simulink model "Q0107tsmc_egtsmc_egftsmc_final_sensitivity"  (R2024b)
settings: Solver=ode4  StartTime=0.0  StopTime=12  FixedStep=0.01  RelTol=1e-3  EnableMultiTasking=on
model workspace (MAT data in the model file):
  A1 = 0.0190784648009
  A2 = 0.089786568484
  B1 = 2.58582251419
  B2 = 0.593361860386
  Count = 20
  I1 = 0.276
  I2 = 0.0235
  I3 = 0.0235
  L1 = 0.5
  L2 = 0.4
  Lp1d = 0.49
  Lp2d = 0.39
  Lp3d = 0.39
  Tmax = 0
  Tmin = -1567
  alpha1 = 1.4711
  alpha2 = 1.4464
  b10 = 33.49
  b11 = 1.435
  b12 = 3.205e-06
  b13 = -161.2
  b14 = 3.294
  b15 = -1.575e-05
  d10 = -0.78
  d11 = -76.79
  d20 = -0.4716
  d21 = 0.47
  dq = [1.72653408644e-22 0.000273900412394 0.000547772970539 0.000821597382973 0.00109535342539 0.0013690210252 0.00164258022129 0.0019160110909 0.00218929391546 0.0024624089498 0.00273533666065 0.00300805756768 ... (1200 elements, 400x3)]
  f10 = 0.0038
  f11 = 141.13
  f20 = 0.0012
  f21 = 150.24
  fai1d = 0.03998
  fai2d = 0.01996
  fai3d = 0.01996
  fce10 = 164.4
  fec11 = 0.003852
  fec12 = -0.9149
  g = 9.8
  ii = -1
  jj = 1
  k10 = 13640
  k11 = 0.05356
  k12 = -37.89
  kk = -1
  ks1 = 394.1176
  ks2 = 379.0476
  ll = 0
  m1 = 3.612
  m2 = 1.762
  nn = 0.1
  out : Simulink.SimulationOutput (value not decoded)
  p0 = 0
  q = [4.04864701555e-21 2.889959974e-21 2.73900412394e-06 8.21673382933e-06 1.64327076591e-05 2.7386241913e-05 4.1076452165e-05 5.75022543779e-05 7.66623652868e-05 9.85553044414e-05 0.000123179393939 0.000150532760546 ... (1200 elements, 400x3)]
  r = 0.05
  rhos0 = 76.79
  rhos1 = -1.54
  rhos2 = 0.4716
  rhos3 = 0.0969
  rhos4 = 78.21
  rhos5 = -1.6
  rhos6 = 0.3214
  rhos7 = 0.0821
  str = 'save 52216121_Testing20_data'
undefined symbols (not defined in the file): A, B, d1, d2, gam1, gam2, ks, kv, q_expanded
libraries: simulink x3, dspswit3 x1
(part 2 of 2)

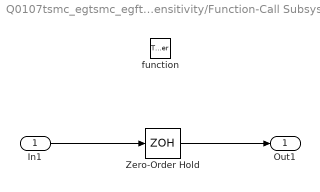
== system Q0107tsmc_egtsmc_egftsmc_final_sensitivity/Function-Call Subsystem2 ==
  In1 : Inport
  function : TriggerPort  VariantControl=Variant
  Zero-Order Hold : ZeroOrderHold  SampleTime=-1
  Out1 : Outport  VectorParamsAs1DForOutWhenUnconnected=off
  wires:
  Zero-Order Hold/1 -> Out1/1
  In1/1 -> Zero-Order Hold/1

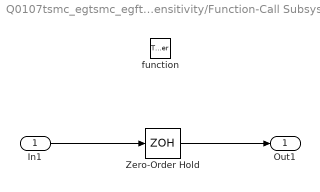
== system Q0107tsmc_egtsmc_egftsmc_final_sensitivity/Function-Call Subsystem3 ==
  In1 : Inport
  function : TriggerPort  VariantControl=Variant
  Zero-Order Hold : ZeroOrderHold  SampleTime=-1
  Out1 : Outport  VectorParamsAs1DForOutWhenUnconnected=off
  wires:
  In1/1 -> Zero-Order Hold/1
  Zero-Order Hold/1 -> Out1/1

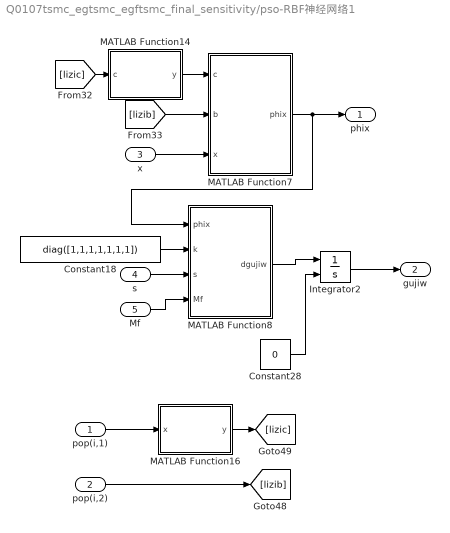
== system Q0107tsmc_egtsmc_egftsmc_final_sensitivity/pso-RBF神经网络1 ==
  pop(i,1) : Inport
  pop(i,2) : Inport  Port=2
  x : Inport  Port=3
  s : Inport  Port=4
  Mf : Inport  Port=5
  Constant18 : Constant  Value=diag([1,1,1,1,1,1,1])
  Constant28 : Constant  Value=0
  Integrator2 : Integrator  InitialConditionSource=external
  MATLAB Function14 : MATLAB Function  TreatAsAtomicUnit=on
  MATLAB Function16 : MATLAB Function  TreatAsAtomicUnit=on
  MATLAB Function7 : MATLAB Function  TreatAsAtomicUnit=on
  MATLAB Function8 : MATLAB Function  TreatAsAtomicUnit=on
  phix : Outport  VectorParamsAs1DForOutWhenUnconnected=off
  gujiw : Outport  Port=2  VectorParamsAs1DForOutWhenUnconnected=off
  wires:
  Integrator2/1 -> gujiw/1
  MATLAB Function8/1(dgujiw) -> Integrator2/1
  s/1 -> MATLAB Function8/3(s)
  Constant28/1 -> Integrator2/2
  x/1 -> MATLAB Function7/3(x)
  [lizib] -> MATLAB Function7/2(b)
  pop(i,1)/1 -> MATLAB Function16/1(x)
  pop(i,2)/1 -> [lizib]
  MATLAB Function16/1(y) -> [lizic]
  MATLAB Function7/1(phix) -> MATLAB Function8/1(phix), phix/1
  Constant18/1 -> MATLAB Function8/2(k)
  [lizic] -> MATLAB Function14/1(c)
  MATLAB Function14/1(y) -> MATLAB Function7/1(c)
  Mf/1 -> MATLAB Function8/4(Mf)

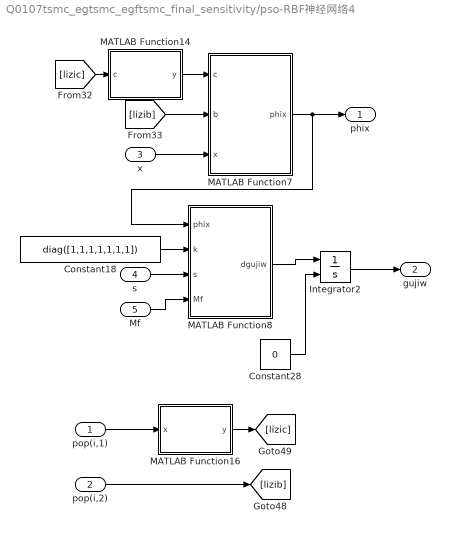
== system Q0107tsmc_egtsmc_egftsmc_final_sensitivity/pso-RBF神经网络4 ==
  pop(i,1) : Inport
  pop(i,2) : Inport  Port=2
  x : Inport  Port=3
  s : Inport  Port=4
  Mf : Inport  Port=5
  Constant18 : Constant  Value=diag([1,1,1,1,1,1,1])
  Constant28 : Constant  Value=0
  Integrator2 : Integrator  InitialConditionSource=external
  MATLAB Function14 : MATLAB Function  TreatAsAtomicUnit=on
  MATLAB Function16 : MATLAB Function  TreatAsAtomicUnit=on
  MATLAB Function7 : MATLAB Function  TreatAsAtomicUnit=on
  MATLAB Function8 : MATLAB Function  TreatAsAtomicUnit=on
  phix : Outport  VectorParamsAs1DForOutWhenUnconnected=off
  gujiw : Outport  Port=2  VectorParamsAs1DForOutWhenUnconnected=off
  wires:
  Mf/1 -> MATLAB Function8/4(Mf)
  MATLAB Function14/1(y) -> MATLAB Function7/1(c)
  [lizic] -> MATLAB Function14/1(c)
  Constant18/1 -> MATLAB Function8/2(k)
  MATLAB Function7/1(phix) -> phix/1, MATLAB Function8/1(phix)
  MATLAB Function16/1(y) -> [lizic]
  pop(i,2)/1 -> [lizib]
  pop(i,1)/1 -> MATLAB Function16/1(x)
  [lizib] -> MATLAB Function7/2(b)
  x/1 -> MATLAB Function7/3(x)
  Constant28/1 -> Integrator2/2
  s/1 -> MATLAB Function8/3(s)
  MATLAB Function8/1(dgujiw) -> Integrator2/1
  Integrator2/1 -> gujiw/1

== matlab function Q0107tsmc_egtsmc_egftsmc_final_sensitivity/Fp1输出1 ==
  data: Uf output; Mf input; Cf input; Gf input; rous input; dx input; ddxd input; s input; ds input; kv input; ks input; d1 input; d2 input; e input; trigger input; last_Uf input; fx input
function Uf = Function(Mf,Cf,Gf,rous, dx, ddxd,s,ds,kv,ks,d1,d2,e,trigger,last_Uf,fx)

Uf=zeros(3,1);



omiga=[abs(s(1))^(d1)*sign(s(1))+abs(s(1))^(d2)*sign(s(1));
    abs(s(2))^(d1)*sign(s(2))+abs(s(2))^(d2)*sign(s(2));
    abs(s(3))^(d1)*sign(s(3))+abs(s(3))^(d2)*sign(s(3));];

oumi=[(ds(1)-rous(1))/rous(1);(ds(2)-rous(2))/rous(2);(ds(3)-rous(3))/rous(3)];

if trigger==1
    Uf=Mf*ddxd+Cf*dx+Gf-Mf*oumi-kv*Mf*tanh(s)-ks*Mf*omiga  ;
else
    Uf=last_Uf;
end

== matlab function Q0107tsmc_egtsmc_egftsmc_final_sensitivity/PrescribedExternalDisturbance ==
  data: t input; dExt output; Uref input; lambda input
function dExt = fcn(t,Uref,lambda)
% Positive dExt is an opposing generalized force in the plant equation.
% Time window: 20%-80% of nominal reference motion, fixed before tests.
ta = 2.36;
tb = 5.65;
r = 0;
if t >= ta && t <= tb
    r = sin(pi*(t-ta)/(tb-ta))^2;
end
dExt = lambda*Uref*r;
end

== matlab function Q0107tsmc_egtsmc_egftsmc_final_sensitivity/MATLAB Function6 ==
  data: Lp1d input; Lp2d input; fai1dd output; Lp3d input; alpha1 input; alpha2 input; alpha3 input; r input; Lx1 input; Lx2 input; Lx3 input; fai2dd output; fai3dd output
function [fai1dd,fai2dd,fai3dd]= fcn(Lp1d,Lp2d,Lp3d,alpha1,alpha2,alpha3,r,Lx1,Lx2,Lx3)




fai1dd = alpha1-acos((r*r+Lx1*Lx1-Lp1d*Lp1d)/2/r/Lx1);
fai2dd = alpha2-acos((r*r+Lx2*Lx2-Lp2d*Lp2d)/2/r/Lx2);
fai3dd = alpha3-acos((r*r+Lx3*Lx3-Lp3d*Lp3d)/2/r/Lx3);

== matlab function Q0107tsmc_egtsmc_egftsmc_final_sensitivity/Lx1 ==
  data: r input; L1 input; Lx1 output; L2 input; L3 input; Lx2 output; Lx3 output
function [Lx1,Lx2,Lx3] = fcn(r,L1,L2,L3)

Lx1 = sqrt(r*r+L1*L1);
Lx2 = sqrt(r*r+L2*L2);
Lx3 = sqrt(r*r+L3*L3);

end

== matlab function Q0107tsmc_egtsmc_egftsmc_final_sensitivity/XBB1 ==
  data: ddxd input; dxd input; xd input; dxB input; xBB output; xB input
function xBB  = fcn(ddxd,dxd,xd,dxB,xB)


xBB=[ddxd',dxd',xd',dxB',xB'];

end

== matlab function Q0107tsmc_egtsmc_egftsmc_final_sensitivity/pso-RBF神经网络1/MATLAB Function14 ==
  data: c input; y output
function y = fcn(c)

y = [c;c;c];

== matlab function Q0107tsmc_egtsmc_egftsmc_final_sensitivity/MATLAB Function5 ==
  data: Lp1d input; Lp2d input; xd output; Lp3d input; t input; yushe input
function xd = fcn(Lp1d,Lp2d,Lp3d,t,yushe)


Lp1dd=0.005*cos(1*t) + Lp1d;
Lp2dd=0.005*cos(1*t) + Lp2d;
Lp3dd=0.005*cos(1*t) + Lp3d;
%xd = [Lp1dd,Lp2dd,Lp3dd]';

%xd = [Lp1d,Lp2d,Lp3d]';

xd=yushe;

%xd=yushe;

== matlab function Q0107tsmc_egtsmc_egftsmc_final_sensitivity/pso-RBF神经网络1/MATLAB Function16 ==
  data: x input; y output
function y = fcn(x)

y = [-x -2*x/3 -x/3 0 x/3 x*2/3 x;
     -x -2*x/3 -x/3 0 x/3 x*2/3 x;
     -x -2*x/3 -x/3 0 x/3 x*2/3 x;
     -x -2*x/3 -x/3 0 x/3 x*2/3 x;
     -x -2*x/3 -x/3 0 x/3 x*2/3 x];

== matlab function Q0107tsmc_egtsmc_egftsmc_final_sensitivity/pso-RBF神经网络1/MATLAB Function7 ==
  data: c input; phix output; b input; x input
function phix = fcn(c,b,x)

phix=zeros(7,1);

for j = 1:1:7
     phix(j) = exp(-norm(x-c(:,j))^2/(b^2));  
end

== matlab function Q0107tsmc_egtsmc_egftsmc_final_sensitivity/pso-RBF神经网络1/MATLAB Function8 ==
  data: phix input; dgujiw output; k input; s input; Mf input
function dgujiw = fcn(phix,k,s,Mf)
dgujiw=zeros(3,7);
dgujiw=(k*phix*s'*pinv(Mf))';

== matlab function Q0107tsmc_egtsmc_egftsmc_final_sensitivity/事件触发条件1 ==
  data: sample_zeta_e input; trigger output; ek output; e input; alpha input; lambda input; Ld input; norm_ek output; threshold output; Lf input; sigma0 input; delta0 input
function [trigger,ek,norm_ek,threshold] = fcn(sample_zeta_e, e, alpha,lambda,Ld,Lf,sigma0,delta0)


trigger=0;



ek=e-sample_zeta_e;


norm_ek = norm(ek);
%threshold = sigma * beta*norm(e) ;
%threshold=alpha/(sqrt(1 + lambda^2) * (lambda + sqrt(2*Ld + 2*Lf)));

threshold = (sigma0 * norm(e) + delta0).^2;

if norm_ek^2 > threshold 
    trigger = 1;
elseif norm_ek^2 < threshold
    trigger = 0;
else
    trigger = 0;
end

== matlab function Q0107tsmc_egtsmc_egftsmc_final_sensitivity/MATLAB Function10 ==
  data: Tmax input; TT output; Tmin input; nn input; T input
function TT = fcn(Tmax,Tmin,nn,T)
Ts=(Tmax+Tmin)/2;
Tp=(Tmax-Tmin)/2;
TT=1/(2*nn)*log(cosh(nn*(T+Tp-Ts))/cosh(nn*(T-Tp-Ts)))+Ts;

== matlab function Q0107tsmc_egtsmc_egftsmc_final_sensitivity/MATLAB Function3 ==
  data: Tmax input; TT output; Tmin input; nn input; T input
function TT = fcn(Tmax,Tmin,nn,T)
Ts=(Tmax+Tmin)/2;
Tp=(Tmax-Tmin)/2;
TT=1/(2*nn)*log(cosh(nn*(T+Tp-Ts))/cosh(nn*(T-Tp-Ts)))+Ts;

== matlab function Q0107tsmc_egtsmc_egftsmc_final_sensitivity/MATLAB Function11 ==
  data: defai2 input; defai3 input; deLp1 input; deLp2 input; deLp3 input; I1 input; I2 input; I3 input; L1 input; L2 input; L3 input; m1 input; m2 input; m3 input; fai1 input; fai2 input; fai3 input; Lp1 input; Lp2 input; Lp3 input; r input; Lx1 input; Lx2 input; Lx3 input; ks1 input; ks2 input; ks3 input; alpha1 input; alpha2 input; alpha3 input; g input; Cf output; Gf output; G1 output; G2 output; G3 output; Mf output; bp1 input; bp2 input; bp3 input; bp4 input; bp5 input; bp6 input; bp7 input; bp8 input; bp9 input; bp10 input; bp11 input; bp12 input; deltaMassInertia input; deltaStiffness input; CfPlant output; GfPlant output; MfPlant output
function [Cf,Gf,G1,G2,G3,Mf,CfPlant,GfPlant,MfPlant] = MATLAB_Function2(defai2,defai3,deLp1,deLp2,deLp3,I1,I2,I3,L1,L2,L3,m1,m2,m3,fai1,fai2,fai3,Lp1,Lp2,Lp3,r,Lx1,Lx2,Lx3,ks1,ks2,ks3,alpha1,alpha2,alpha3,g,bp1,bp2,bp3,bp4,bp5,bp6,bp7,bp8,bp9,bp10,bp11,bp12,deltaMassInertia,deltaStiffness)
% Controller uses nominal matrices. Plant matrices come from perturbed physical parameters.
% Retains the original dynamics implementation, including M21=M11.
[Cf,Gf,G1,G2,G3,Mf] = localDynamics(defai2,defai3,deLp1,deLp2,deLp3,I1,I2,I3,L1,L2,L3,m1,m2,m3,fai1,fai2,fai3,Lp1,Lp2,Lp3,r,Lx1,Lx2,Lx3,ks1,ks2,ks3,alpha1,alpha2,alpha3,g,bp1,bp2,bp3,bp4,bp5,bp6,bp7,bp8,bp9,bp10,bp11,bp12);
[CfPlant,GfPlant,~,~,~,MfPlant] = localDynamics(defai2,defai3,deLp1,deLp2,deLp3,I1*(1+deltaMassInertia),I2*(1+deltaMassInertia),I3*(1+deltaMassInertia),L1,L2,L3,m1*(1+deltaMassInertia),m2*(1+deltaMassInertia),m3*(1+deltaMassInertia),fai1,fai2,fai3,Lp1,Lp2,Lp3,r,Lx1,Lx2,Lx3,ks1*(1+deltaStiffness),ks2*(1+deltaStiffness),ks3*(1+deltaStiffness),alpha1,alpha2,alpha3,g,bp1,bp2,bp3,bp4,bp5,bp6,bp7,bp8,bp9,bp10,bp11,bp12);
end

function [Cf,Gf,G1,G2,G3,Mf] = localDynamics(defai2,defai3,deLp1,deLp2,deLp3,I1,I2,I3,L1,L2,L3,m1,m2,m3,fai1,fai2,fai3,Lp1,Lp2,Lp3,r,Lx1,Lx2,Lx3,ks1,ks2,ks3,alpha1,alpha2,alpha3,g,bp1,bp2,bp3,bp4,bp5,bp6,bp7,bp8,bp9,bp10,bp11,bp12)
ac1=r*r+Lx1*Lx1;
ac3=r*r+Lx2*Lx2;
ac5=r*r+Lx3*Lx3;


up1=I1+I2+I3+m2*(L1*L1+0.25*L2*L2+L1*L2*cos(fai2))+m3*(L1*L1+L2*L2+0.25*L3*L3+2*L1*L2*cos(fai2)+L2*L3*cos(fai3)+L1*L3*cos(fai3+fai2));
up2=I2+I3+0.25*m2*L2*L2+m3*(L2*L2+0.25*L3*L3+L2*L3*cos(fai3));
up3=I3+0.25*m3*L3*L3;
up4=I2+I3+0.5*m2*(0.5*L2*L2+L1*L2*cos(fai2))+0.5*m3*(2*L2*L2+0.5*L3*L3+2*L1*L2*cos(fai2)+2*L2*L3*cos(fai3)+L1*L3*cos(fai3+fai2));
up5=I3+0.5*m3*(0.5*L3*L3+L2*L3*cos(fai3));
up6=I3+0.5*m3*(0.5*L3*L3+L2*L3*cos(fai3)+L1*L3*cos(fai2+fai3));
up7=r*r+Lx1*Lx1-2*r*Lx1*cos(fai1+alpha1);
up8=r*r+Lx2*Lx2-2*r*Lx2*cos(fai2+alpha2);
up9=r*r+Lx3*Lx3-2*r*Lx3*cos(fai3+alpha3);
up11=4*Lx1*Lx1*r*r-(r*r+Lx1^2-Lp1^2)^2;
up21=4*Lx2*Lx2*r*r-(r*r+Lx2^2-Lp2^2)^2;
up31=4*Lx3*Lx3*r*r-(r*r+Lx3^2-Lp3^2)^2;


C11 = -(m2*L1*L2*defai2*sin(fai2)+2*m3*L1*L2*defai2*sin(fai2)+m3*L2*L3*defai3*sin(fai3)+m3*L1*L3*(defai2+defai3)*sin(fai2+fai3))*2*Lp1*Lp1/up11 ...
+4*up1*Lp1*deLp1/up11-8*(r*r+Lx1*Lx1)*up1*Lp1^3*deLp1/up11/up11+8*up1*(Lp1^5)*deLp1/up11/up11;

C12=(2*m2*L1*L2*sin(fai2)+4*m3*L1*L2*sin(fai2)+4*m3*L2*L3*sin(fai3)+2*m3*L1*L3*sin(fai2+fai3))*Lp1*Lp1*deLp1*Lp2/up11/sqrt((up21)) ...
+(2*m2*L1*L2*sin(fai2)+4*m3*L1*L2*sin(fai2)+4*m3*L2*L3*sin(fai3)+2*m3*L1*L3*sin(fai2+fai3))*Lp1*deLp2*Lp2*Lp2/up21/sqrt((up11))...
+4*up4*Lp1*deLp2/sqrt((up11*up21))-8*up4*((r*r+Lx2*Lx2)*Lp2-Lp2^3)*Lp1*Lp2*deLp2/up21/sqrt((up11*up21));

C13=(2*m3*L2*L3*sin(fai3)+2*m3*L1*L3*sin(fai2+fai3))*Lp1*Lp1*deLp1*Lp3/up11/sqrt((up31)) ...
+(2*m3*L2*L3*sin(fai3)+2*m3*L1*L3*sin(fai2+fai3))*Lp1*Lp3*Lp3*deLp3/up31/sqrt((up11))...
+4*up6*Lp1*deLp3/sqrt((up11*up31))-8*up6*((r*r+Lx3*Lx3)*Lp3-Lp3^3)*Lp1*Lp3*deLp3/up31/sqrt((up11*up31));

C21=-(2*m2*L1*L2*defai2*sin(fai2)+4*m3*L1*L2*defai2*sin(fai2)+4*m3*L2*L3*defai3*sin(fai3)+2*m3*L1*L3*(defai2+defai3)*sin(fai2+fai3))*Lp1*Lp2/sqrt((up11*up21)) ...
-(2*m2*L1*L2*sin(fai2)+4*m3*L1*L2*sin(fai2)+4*m3*L2*L3*sin(fai3)+2*m3*L1*L3*sin(fai2+fai3))*Lp1*Lp2*Lp2*deLp2/up21/sqrt((up11))...
-(2*m2*L1*L2*sin(fai2)+4*m3*L1*L2*sin(fai2)+4*m3*L2*L3*sin(fai3)+2*m3*L1*L3*sin(fai2+fai3))*Lp1*Lp1*Lp2*deLp1/up11/sqrt((up21))...
+4*up4*deLp1*Lp2/sqrt((up11*up21))-8*up4*((r*r+Lx1*Lx1)*Lp1-Lp1^3)*Lp1*Lp2*deLp1/up11/sqrt((up11*up21));

C22=-m3*L2*L3*defai3*sin(fai3)*2*Lp2*Lp2/up21+4*up2*Lp2*deLp2/up21-8*(r*r+Lx2*Lx2)*up2*Lp2*Lp2*Lp2*deLp2/up21/up21+8*up2*(Lp2^5)*deLp2/up21/up21;

C23=2*m3*L2*L3*sin(fai3)*Lp2*Lp3*Lp3*deLp3/up31/sqrt((up21))+2*m3*L2*L3*sin(fai3)*Lp2*Lp2*Lp3*deLp2/up21/sqrt((up31))...
+4*up5*Lp2*deLp3/sqrt((up21*up31))-8*up5*((r*r+Lx3*Lx3)*Lp3-Lp3^3)*Lp2*Lp3*deLp3/up31/sqrt((up31*up21));

C31=-(2*m3*L2*L3*defai3*sin(fai3)+2*m3*L1*L3*(defai2+defai3)*sin(fai2+fai3))*Lp1*Lp3/sqrt((up11*up31)) ...
-(2*m3*L2*L3*sin(fai3)+2*m3*L1*L3*sin(fai2+fai3))*Lp1*Lp3*Lp3*deLp3/up31/sqrt((up11))...
-(2*m3*L2*L3*sin(fai3)+2*m3*L1*L3*sin(fai2+fai3))*Lp1*Lp1*deLp1*Lp3/up11/sqrt((up31))...
+4*up6*Lp3*deLp1/sqrt((up11*up31))-8*up6*((r*r+Lx1*Lx1)*Lp1-Lp1^3)*Lp1*Lp3*deLp1/up11/sqrt((up31*up11));

C32=-2*m3*L2*L3*defai3*sin(fai3)*Lp2*Lp3/sqrt((up21*up31))-2*m3*L2*L3*sin(fai3)*Lp2*Lp2*deLp2*Lp3/up21/sqrt((up31)) ...
-2*m3*L2*L3*sin(fai3)*Lp2*Lp3*deLp3*Lp3/up31/sqrt((up21))+4*up5*deLp2*Lp3/sqrt((up21*up31))-8*up5*((r*r+Lx2*Lx2)*Lp2-Lp2^3)*Lp2*Lp3*deLp2/up21/sqrt((up31*up21));

C33=4*up3*Lp3*deLp3/up31-8*up3*(r*r+Lx3*Lx3)*Lp3*Lp3*Lp3*deLp3/up31/up31+8*up3*(Lp3^5)*deLp3/up31/up31;

G1=-m1*g*L1*sin(fai1)*Lp1/sqrt((up11))-m2*g*(L1*sin(fai1)+0.5*L2*sin(fai1+fai2))*Lp1/sqrt((up11)) ...
-2*m3*g*(L1*sin(fai1)+L2*sin(fai1+fai2)+0.5*L3*sin(fai1+fai2+fai3))*Lp1/sqrt((up11))...
-2*ks1*r*Lx1*Lp1*sin(fai1+alpha1)*(sqrt((up7))-L1)/sqrt((up11*up7));

G2=-m2*g*L2*sin(fai1+fai2)*Lp2/sqrt((up21))-2*m3*g*(L2*sin(fai1+fai2)+0.5*L3*sin(fai1+fai2+fai3))*Lp2/sqrt((up21)) ...
-2*ks2*r*Lx2*Lp2*sin(fai2+alpha2)*(sqrt((up8))-L2)/sqrt((up21*up8));

G3=-m3*g*L3*sin(fai1+fai2+fai3)*Lp3/sqrt((up31))-2*ks3*r*Lx3*Lp3*sin(fai3+alpha3)*(sqrt((up9))-L3)/sqrt((up31*up9));




M11=4*up1*Lp1*Lp1/up11;
M12=4*up4*Lp1*Lp2/sqrt(abs(up11*up21));M21=M11;
M23=4*up5*Lp3*Lp2/sqrt(abs(up21*up31));M32=M23;
M13=4*up6*Lp1*Lp3/sqrt(abs(up11*up31));M31=M13;
M22=4*up2*Lp2*Lp2/up21;
M33=4*up3*Lp3*Lp3/up31;

M41=2*Lp1/sqrt(abs(up11));
M52=2*Lp2/sqrt(abs(up21));
M63=2*Lp3/sqrt(abs(up31));
C41=2*deLp1/sqrt(abs(up11))-4*Lp1*deLp1*(ac1*Lp1-Lp1*Lp1*Lp1)/up11/sqrt(abs(up11));
C52=2*deLp2/sqrt(abs(up21))-4*Lp2*deLp2*(ac3*Lp2-Lp2*Lp2*Lp2)/up21/sqrt(abs(up21));
C63=2*deLp3/sqrt(abs(up31))-4*Lp3*deLp3*(ac5*Lp3-Lp3*Lp3*Lp3)/up31/sqrt(abs(up31));



Cf = [C11+bp4 C12 C13 ;
    C21 C22+bp5 C23 ;
    C31 C32 C33+bp6 ;
 ];


Mf = [M11 M12 M13 ;
    M21 M22 M23 ;
    M31 M32 M33 ;
];


Gf = [G1+bp1+bp7*Lp1-bp10*Lp1*Lp1;
    G2+bp2+bp8*Lp2-bp11*Lp2*Lp2;
    G3+bp3+bp9*Lp3-bp12*Lp3*Lp3;
    ];
end

== matlab function Q0107tsmc_egtsmc_egftsmc_final_sensitivity/MATLAB Function9 ==
  data: Tmax input; TT output; Tmin input; nn input; T input
function TT = fcn(Tmax,Tmin,nn,T)
Ts=(Tmax+Tmin)/2;
Tp=(Tmax-Tmin)/2;
TT=1/(2*nn)*log(cosh(nn*(T+Tp-Ts))/cosh(nn*(T-Tp-Ts)))+Ts;

== matlab function Q0107tsmc_egtsmc_egftsmc_final_sensitivity/滑模面2 ==
  data: e input; s output; de input; ie input; A input; B input; C input; gam1 input; gam2 input; rous output
function [s,rous]= fcn(e,de,ie,A,B,C,gam1,gam2)



s1=tanh(e(1))+A*abs(tanh(e(1)))^gam1*sign(e(1))+B*(1-(tanh(e(1))^2))^gam2*abs(de(1))^gam2*sign(de(1));
s2=tanh(e(2))+A*abs(tanh(e(2)))^gam1*sign(e(2))+B*(1-(tanh(e(2))^2))^gam2*abs(de(2))^gam2*sign(de(2));
s3=tanh(e(3))+A*abs(tanh(e(3)))^gam1*sign(e(3))+B*(1-(tanh(e(3))^2))^gam2*abs(de(3))^gam2*sign(de(3));

rous1=gam2*B*(1-tanh(e(1))^2)^gam2*abs(de(1))^(gam2-1);
rous2=gam2*B*(1-tanh(e(2))^2)^gam2*abs(de(2))^(gam2-1);
rous3=gam2*B*(1-tanh(e(3))^2)^gam2*abs(de(3))^(gam2-1);

rous=[rous1;rous2;rous3];


s=[s1;
   s2;
   s3];

== matlab function Q0107tsmc_egtsmc_egftsmc_final_sensitivity/Fp1输出4 ==
  data: fx input; Uf output; Mf input; Cf input; Gf input; rous input; dx input; ddxd input; s input; ds input; kv input; ks input; d1 input; d2 input
function Uf = Function(fx,Mf,Cf,Gf,rous, dx, ddxd,s,ds,kv,ks,d1,d2)

Uf=zeros(3,1);



omiga=[abs(s(1))^(d1)*sign(s(1))+abs(s(1))^(d2)*sign(s(1));
    abs(s(2))^(d1)*sign(s(2))+abs(s(2))^(d2)*sign(s(2));
    abs(s(3))^(d1)*sign(s(3))+abs(s(3))^(d2)*sign(s(3));];

oumi=[(ds(1)-rous(1))/rous(1);(ds(2)-rous(2))/rous(2);(ds(3)-rous(3))/rous(3)];

Uf=Mf*ddxd+Cf*dx+Gf-Mf*oumi-kv*Mf*tanh(s)-ks*Mf*omiga  ;

%Uf=fx-kv*Mf*tanh(s)-ks*Mf*omiga;







end

== matlab function Q0107tsmc_egtsmc_egftsmc_final_sensitivity/lambc1 ==
  data: Lp1 input; Lp2 input; Lp3 input; L1 input; L2 input; L3 input; f10 input; f11 input; f20 input; f21 input; f30 input; f31 input; rhos0 input; rhos1 input; rhos2 input; rhos3 input; rhos4 input; rhos5 input; rhos6 input; rhos7 input; rhos8 input; rhos9 input; rhos10 input; rhos11 input; p0 input; d10 input; d11 input; d20 input; d21 input; d30 input; d31 input; Os output size=[3 1]; U output size=[3 1]; Uf input; bp1 output; bp2 output; bp3 output; bp4 output; bp5 output; bp6 output; bp7 output; bp8 output; bp9 output; bp10 output; bp11 output; bp12 output; B1 output; B2 output
function [Os,U,bp1,bp2,bp3,bp4,bp5,bp6,bp7,bp8,bp9,bp10,bp11,bp12,B1,B2]= fcn(Lp1,Lp2,Lp3,L1,L2,L3,f10,f11,f20,f21,f30,f31, ...
    rhos0,rhos1,rhos2,rhos3,rhos4,rhos5,rhos6,rhos7,rhos8,rhos9,rhos10,rhos11,p0,d10,d11,d20,d21,d30,d31,Uf)

bp1=f11*p0+f10-(rhos1*p0+rhos0)*L1-(rhos3*p0+rhos2)*L1*L1;
bp2=f21*p0+f20-(rhos5*p0+rhos4)*L2-(rhos7*p0+rhos6)*L2*L2;
bp3=f31*p0+f30-(rhos9*p0+rhos8)*L3-(rhos11*p0+rhos10)*L3*L3;
bp4=d11*p0+d10;
bp5=d21*p0+d20;
bp6=d31*p0+d30;
bp7=rhos1*p0+rhos0+2*L1*(rhos3*p0+rhos2);
bp8=rhos5*p0+rhos4+2*L2*(rhos7*p0+rhos6);
bp9=rhos9*p0+rhos8+2*L3*(rhos11*p0+rhos10);
bp10=rhos3*p0+rhos2;
bp11=rhos7*p0+rhos6;
bp12=rhos11*p0+rhos10;


lambc1 = rhos1*Lp1-rhos3*(Lp1*Lp1-2*L1*Lp1);
lambc2 = rhos5*Lp2-rhos7*(Lp2*Lp2-2*L2*Lp2);
lambc3 = rhos9*Lp3-rhos11*(Lp3*Lp3-2*L3*Lp3);

B1 = [lambc1 0 0 ;
    0 lambc2 0 ;
    0 0 lambc3];

lambs1 = f11-rhos1*L1-rhos3*L1*L1;
lambs2 = f21-rhos5*L2-rhos7*L2*L2;
lambs3 = f31-rhos9*L3-rhos11*L3*L3;

B2 = [-lambs1 0 0 ;
    0 -lambs2 0 ;
    0 0 -lambs3 ];


U = pinv(B2)*Uf;


Os = B1*U;

end

== matlab function Q0107tsmc_egtsmc_egftsmc_final_sensitivity/Lx2 ==
  data: r input; Lx1 input; Lx2 input; Lx3 input; fai1 output; alpha1 input; alpha2 input; alpha3 input; Lp1 input; Lp2 input; Lp3 input; fai2 output; fai3 output
function [fai1,fai2,fai3] = fcn(r,Lx1,Lx2,Lx3,alpha1,alpha2,alpha3,Lp1,Lp2,Lp3)



fai1=alpha1-acos((r*r+Lx1*Lx1-Lp1*Lp1)/2/r/Lx1);
fai2=alpha2-acos((r*r+Lx2*Lx2-Lp2*Lp2)/2/r/Lx2);
fai3=alpha3-acos((r*r+Lx3*Lx3-Lp3*Lp3)/2/r/Lx3);

end

== matlab function Q0107tsmc_egtsmc_egftsmc_final_sensitivity/Lx4 ==
  data: r input; Lx1 input; Lx2 input; Lx3 input; fai1 output; alpha1 input; alpha2 input; alpha3 input; Lp1 input; Lp2 input; Lp3 input; fai2 output; fai3 output
function [fai1,fai2,fai3] = fcn(r,Lx1,Lx2,Lx3,alpha1,alpha2,alpha3,Lp1,Lp2,Lp3)



fai1=alpha1-acos((r*r+Lx1*Lx1-Lp1*Lp1)/2/r/Lx1);
fai2=alpha2-acos((r*r+Lx2*Lx2-Lp2*Lp2)/2/r/Lx2);
fai3=alpha3-acos((r*r+Lx3*Lx3-Lp3*Lp3)/2/r/Lx3);

end

== matlab function Q0107tsmc_egtsmc_egftsmc_final_sensitivity/MATLAB Function12 ==
  data: Mf input; Uf input; ddx output; Cf input; dx input; Gf input; Os input; dExt input
function ddx = fcn(Mf,Uf,Cf,dx,Gf,Os,dExt)
% Controller does not receive dExt. Positive dExt opposes negative PAM force.
ddx = pinv(Mf)*(Uf-Cf*dx-Gf-Os+dExt);
end

== matlab function Q0107tsmc_egtsmc_egftsmc_final_sensitivity/MATLAB Function13 ==
  data: lambc1 input; lambc2 input; lambc3 input; lambs1 input; lambs2 input; Fp output; lambs3 input; p input; Lp1 input; Lp2 input; Lp3 input; dLp1 input; dLp2 input; dLp3 input; bp1 input; bp2 input; bp3 input; bp4 input; bp5 input; bp6 input; bp7 input; bp8 input; bp9 input; bp10 input; bp11 input; bp12 input
function Fp = fcn(lambc1,lambc2,lambc3,lambs1,lambs2,lambs3,p,Lp1,Lp2,Lp3,dLp1,dLp2,dLp3, ...
    bp1,bp2,bp3,bp4,bp5,bp6,bp7,bp8,bp9,bp10,bp11,bp12)


Fp1=lambs1*p(1)+lambc1*p(1)+bp1+bp4*dLp1+bp7*Lp1-bp10*Lp1^2;
Fp2=lambs2*p(2)+lambc2*p(2)+bp2+bp5*dLp2+bp8*Lp2-bp11*Lp2^2;
Fp3=lambs3*p(3)+lambc3*p(3)+bp3+bp6*dLp3+bp9*Lp3-bp12*Lp3^2;

Fp=[Fp1;Fp2;Fp3];

== matlab function Q0107tsmc_egtsmc_egftsmc_final_sensitivity/计算Lpi2 ==
  data: Mf input; Uf input; ddx output; Cf input; dx input; Gf input; Os input; dExt input
function ddx = fcn(Mf,Uf,Cf,dx,Gf,Os,dExt)
% Controller does not receive dExt. Positive dExt opposes negative PAM force.
ddx = pinv(Mf)*(Uf-Cf*dx-Gf-Os+dExt);
end

== matlab function Q0107tsmc_egtsmc_egftsmc_final_sensitivity/MATLAB Function16 ==
  data: dLp1 input; dLp2 input; dLp3 input; bp4 input; bp5 input; bp6 input; Gf input; B1 input; B2 input; P input; Fp output; G1 input; G2 input; G3 input
function Fp = fcn(dLp1,dLp2,dLp3,bp4,bp5,bp6,Gf,B1,B2,P,G1,G2,G3)


Fp1=B2(1,1)*P(1)-(bp4*dLp1+Gf(1)+B1(1,1)*P(1))+G1;
Fp2=B2(2,2)*P(2)-(bp5*dLp2+Gf(2)+B1(2,2)*P(2))+G2;
Fp3=B2(3,3)*P(3)-(bp6*dLp3+Gf(3)+B1(3,3)*P(3))+G3;

Fp=[Fp1;Fp2;Fp3];

== matlab function Q0107tsmc_egtsmc_egftsmc_final_sensitivity/MATLAB Function14 ==
  data: defai2 input; defai3 input; deLp1 input; deLp2 input; deLp3 input; I1 input; I2 input; I3 input; L1 input; L2 input; L3 input; m1 input; m2 input; m3 input; fai1 input; fai2 input; fai3 input; Lp1 input; Lp2 input; Lp3 input; r input; Lx1 input; Lx2 input; Lx3 input; ks1 input; ks2 input; ks3 input; alpha1 input; alpha2 input; alpha3 input; g input; Cf output; Gf output; Mf output; bp1 input; bp2 input; bp3 input; bp4 input; bp5 input; bp6 input; bp7 input; bp8 input; bp9 input; bp10 input; bp11 input; bp12 input; deltaMassInertia input; deltaStiffness input; CfPlant output; GfPlant output; MfPlant output
function [Cf,Gf,Mf,CfPlant,GfPlant,MfPlant] = MATLAB_Function2(defai2,defai3,deLp1,deLp2,deLp3,I1,I2,I3,L1,L2,L3,m1,m2,m3,fai1,fai2,fai3,Lp1,Lp2,Lp3,r,Lx1,Lx2,Lx3,ks1,ks2,ks3,alpha1,alpha2,alpha3,g,bp1,bp2,bp3,bp4,bp5,bp6,bp7,bp8,bp9,bp10,bp11,bp12,deltaMassInertia,deltaStiffness)
% Controller uses nominal matrices. Plant matrices come from perturbed physical parameters.
% Retains the original dynamics implementation, including M21=M11.
[Cf,Gf,Mf] = localDynamics(defai2,defai3,deLp1,deLp2,deLp3,I1,I2,I3,L1,L2,L3,m1,m2,m3,fai1,fai2,fai3,Lp1,Lp2,Lp3,r,Lx1,Lx2,Lx3,ks1,ks2,ks3,alpha1,alpha2,alpha3,g,bp1,bp2,bp3,bp4,bp5,bp6,bp7,bp8,bp9,bp10,bp11,bp12);
[CfPlant,GfPlant,MfPlant] = localDynamics(defai2,defai3,deLp1,deLp2,deLp3,I1*(1+deltaMassInertia),I2*(1+deltaMassInertia),I3*(1+deltaMassInertia),L1,L2,L3,m1*(1+deltaMassInertia),m2*(1+deltaMassInertia),m3*(1+deltaMassInertia),fai1,fai2,fai3,Lp1,Lp2,Lp3,r,Lx1,Lx2,Lx3,ks1*(1+deltaStiffness),ks2*(1+deltaStiffness),ks3*(1+deltaStiffness),alpha1,alpha2,alpha3,g,bp1,bp2,bp3,bp4,bp5,bp6,bp7,bp8,bp9,bp10,bp11,bp12);
end

function [Cf,Gf,Mf] = localDynamics(defai2,defai3,deLp1,deLp2,deLp3,I1,I2,I3,L1,L2,L3,m1,m2,m3,fai1,fai2,fai3,Lp1,Lp2,Lp3,r,Lx1,Lx2,Lx3,ks1,ks2,ks3,alpha1,alpha2,alpha3,g,bp1,bp2,bp3,bp4,bp5,bp6,bp7,bp8,bp9,bp10,bp11,bp12)
ac1=r*r+Lx1*Lx1;
ac3=r*r+Lx2*Lx2;
ac5=r*r+Lx3*Lx3;


up1=I1+I2+I3+m2*(L1*L1+0.25*L2*L2+L1*L2*cos(fai2))+m3*(L1*L1+L2*L2+0.25*L3*L3+2*L1*L2*cos(fai2)+L2*L3*cos(fai3)+L1*L3*cos(fai3+fai2));
up2=I2+I3+0.25*m2*L2*L2+m3*(L2*L2+0.25*L3*L3+L2*L3*cos(fai3));
up3=I3+0.25*m3*L3*L3;
up4=I2+I3+0.5*m2*(0.5*L2*L2+L1*L2*cos(fai2))+0.5*m3*(2*L2*L2+0.5*L3*L3+2*L1*L2*cos(fai2)+2*L2*L3*cos(fai3)+L1*L3*cos(fai3+fai2));
up5=I3+0.5*m3*(0.5*L3*L3+L2*L3*cos(fai3));
up6=I3+0.5*m3*(0.5*L3*L3+L2*L3*cos(fai3)+L1*L3*cos(fai2+fai3));
up7=r*r+Lx1*Lx1-2*r*Lx1*cos(fai1+alpha1);
up8=r*r+Lx2*Lx2-2*r*Lx2*cos(fai2+alpha2);
up9=r*r+Lx3*Lx3-2*r*Lx3*cos(fai3+alpha3);
up11=4*Lx1*Lx1*r*r-(r*r+Lx1^2-Lp1^2)^2;
up21=4*Lx2*Lx2*r*r-(r*r+Lx2^2-Lp2^2)^2;
up31=4*Lx3*Lx3*r*r-(r*r+Lx3^2-Lp3^2)^2;


C11 = -(m2*L1*L2*defai2*sin(fai2)+2*m3*L1*L2*defai2*sin(fai2)+m3*L2*L3*defai3*sin(fai3)+m3*L1*L3*(defai2+defai3)*sin(fai2+fai3))*2*Lp1*Lp1/up11 ...
+4*up1*Lp1*deLp1/up11-8*(r*r+Lx1*Lx1)*up1*Lp1^3*deLp1/up11/up11+8*up1*(Lp1^5)*deLp1/up11/up11;

C12=(2*m2*L1*L2*sin(fai2)+4*m3*L1*L2*sin(fai2)+4*m3*L2*L3*sin(fai3)+2*m3*L1*L3*sin(fai2+fai3))*Lp1*Lp1*deLp1*Lp2/up11/sqrt((up21)) ...
+(2*m2*L1*L2*sin(fai2)+4*m3*L1*L2*sin(fai2)+4*m3*L2*L3*sin(fai3)+2*m3*L1*L3*sin(fai2+fai3))*Lp1*deLp2*Lp2*Lp2/up21/sqrt((up11))...
+4*up4*Lp1*deLp2/sqrt((up11*up21))-8*up4*((r*r+Lx2*Lx2)*Lp2-Lp2^3)*Lp1*Lp2*deLp2/up21/sqrt((up11*up21));

C13=(2*m3*L2*L3*sin(fai3)+2*m3*L1*L3*sin(fai2+fai3))*Lp1*Lp1*deLp1*Lp3/up11/sqrt((up31)) ...
+(2*m3*L2*L3*sin(fai3)+2*m3*L1*L3*sin(fai2+fai3))*Lp1*Lp3*Lp3*deLp3/up31/sqrt((up11))...
+4*up6*Lp1*deLp3/sqrt((up11*up31))-8*up6*((r*r+Lx3*Lx3)*Lp3-Lp3^3)*Lp1*Lp3*deLp3/up31/sqrt((up11*up31));

C21=-(2*m2*L1*L2*defai2*sin(fai2)+4*m3*L1*L2*defai2*sin(fai2)+4*m3*L2*L3*defai3*sin(fai3)+2*m3*L1*L3*(defai2+defai3)*sin(fai2+fai3))*Lp1*Lp2/sqrt((up11*up21)) ...
-(2*m2*L1*L2*sin(fai2)+4*m3*L1*L2*sin(fai2)+4*m3*L2*L3*sin(fai3)+2*m3*L1*L3*sin(fai2+fai3))*Lp1*Lp2*Lp2*deLp2/up21/sqrt((up11))...
-(2*m2*L1*L2*sin(fai2)+4*m3*L1*L2*sin(fai2)+4*m3*L2*L3*sin(fai3)+2*m3*L1*L3*sin(fai2+fai3))*Lp1*Lp1*Lp2*deLp1/up11/sqrt((up21))...
+4*up4*deLp1*Lp2/sqrt((up11*up21))-8*up4*((r*r+Lx1*Lx1)*Lp1-Lp1^3)*Lp1*Lp2*deLp1/up11/sqrt((up11*up21));

C22=-m3*L2*L3*defai3*sin(fai3)*2*Lp2*Lp2/up21+4*up2*Lp2*deLp2/up21-8*(r*r+Lx2*Lx2)*up2*Lp2*Lp2*Lp2*deLp2/up21/up21+8*up2*(Lp2^5)*deLp2/up21/up21;

C23=2*m3*L2*L3*sin(fai3)*Lp2*Lp3*Lp3*deLp3/up31/sqrt((up21))+2*m3*L2*L3*sin(fai3)*Lp2*Lp2*Lp3*deLp2/up21/sqrt((up31))...
+4*up5*Lp2*deLp3/sqrt((up21*up31))-8*up5*((r*r+Lx3*Lx3)*Lp3-Lp3^3)*Lp2*Lp3*deLp3/up31/sqrt((up31*up21));

C31=-(2*m3*L2*L3*defai3*sin(fai3)+2*m3*L1*L3*(defai2+defai3)*sin(fai2+fai3))*Lp1*Lp3/sqrt((up11*up31)) ...
-(2*m3*L2*L3*sin(fai3)+2*m3*L1*L3*sin(fai2+fai3))*Lp1*Lp3*Lp3*deLp3/up31/sqrt((up11))...
-(2*m3*L2*L3*sin(fai3)+2*m3*L1*L3*sin(fai2+fai3))*Lp1*Lp1*deLp1*Lp3/up11/sqrt((up31))...
+4*up6*Lp3*deLp1/sqrt((up11*up31))-8*up6*((r*r+Lx1*Lx1)*Lp1-Lp1^3)*Lp1*Lp3*deLp1/up11/sqrt((up31*up11));

C32=-2*m3*L2*L3*defai3*sin(fai3)*Lp2*Lp3/sqrt((up21*up31))-2*m3*L2*L3*sin(fai3)*Lp2*Lp2*deLp2*Lp3/up21/sqrt((up31)) ...
-2*m3*L2*L3*sin(fai3)*Lp2*Lp3*deLp3*Lp3/up31/sqrt((up21))+4*up5*deLp2*Lp3/sqrt((up21*up31))-8*up5*((r*r+Lx2*Lx2)*Lp2-Lp2^3)*Lp2*Lp3*deLp2/up21/sqrt((up31*up21));

C33=4*up3*Lp3*deLp3/up31-8*up3*(r*r+Lx3*Lx3)*Lp3*Lp3*Lp3*deLp3/up31/up31+8*up3*(Lp3^5)*deLp3/up31/up31;

G1=-m1*g*L1*sin(fai1)*Lp1/sqrt((up11))-m2*g*(L1*sin(fai1)+0.5*L2*sin(fai1+fai2))*Lp1/sqrt((up11)) ...
-2*m3*g*(L1*sin(fai1)+L2*sin(fai1+fai2)+0.5*L3*sin(fai1+fai2+fai3))*Lp1/sqrt((up11))...
-2*ks1*r*Lx1*Lp1*sin(fai1+alpha1)*(sqrt((up7))-L1)/sqrt((up11*up7));

G2=-m2*g*L2*sin(fai1+fai2)*Lp2/sqrt((up21))-2*m3*g*(L2*sin(fai1+fai2)+0.5*L3*sin(fai1+fai2+fai3))*Lp2/sqrt((up21)) ...
-2*ks2*r*Lx2*Lp2*sin(fai2+alpha2)*(sqrt((up8))-L2)/sqrt((up21*up8));

G3=-m3*g*L3*sin(fai1+fai2+fai3)*Lp3/sqrt((up31))-2*ks3*r*Lx3*Lp3*sin(fai3+alpha3)*(sqrt((up9))-L3)/sqrt((up31*up9));




M11=4*up1*Lp1*Lp1/up11;
M12=4*up4*Lp1*Lp2/sqrt(abs(up11*up21));M21=M11;
M23=4*up5*Lp3*Lp2/sqrt(abs(up21*up31));M32=M23;
M13=4*up6*Lp1*Lp3/sqrt(abs(up11*up31));M31=M13;
M22=4*up2*Lp2*Lp2/up21;
M33=4*up3*Lp3*Lp3/up31;

M41=2*Lp1/sqrt(abs(up11));
M52=2*Lp2/sqrt(abs(up21));
M63=2*Lp3/sqrt(abs(up31));
C41=2*deLp1/sqrt(abs(up11))-4*Lp1*deLp1*(ac1*Lp1-Lp1*Lp1*Lp1)/up11/sqrt(abs(up11));
C52=2*deLp2/sqrt(abs(up21))-4*Lp2*deLp2*(ac3*Lp2-Lp2*Lp2*Lp2)/up21/sqrt(abs(up21));
C63=2*deLp3/sqrt(abs(up31))-4*Lp3*deLp3*(ac5*Lp3-Lp3*Lp3*Lp3)/up31/sqrt(abs(up31));



Cf = [C11+bp4 C12 C13 ;
    C21 C22+bp5 C23 ;
    C31 C32 C33+bp6 ;
 ];


Mf = [M11 M12 M13 ;
    M21 M22 M23 ;
    M31 M32 M33 ;
];


Gf = [G1+bp1+bp7*Lp1-bp10*Lp1*Lp1;
    G2+bp2+bp8*Lp2-bp11*Lp2*Lp2;
    G3+bp3+bp9*Lp3-bp12*Lp3*Lp3;
    ];
end

== matlab function Q0107tsmc_egtsmc_egftsmc_final_sensitivity/MATLAB Function18 ==
  data: Tmax input; TT output; Tmin input; nn input; T input
function TT = fcn(Tmax,Tmin,nn,T)
Ts=(Tmax+Tmin)/2;
Tp=(Tmax-Tmin)/2;
TT=1/(2*nn)*log(cosh(nn*(T+Tp-Ts))/cosh(nn*(T-Tp-Ts)))+Ts;

== matlab function Q0107tsmc_egtsmc_egftsmc_final_sensitivity/MATLAB Function19 ==
  data: Tmax input; TT output; Tmin input; nn input; T input
function TT = fcn(Tmax,Tmin,nn,T)
Ts=(Tmax+Tmin)/2;
Tp=(Tmax-Tmin)/2;
TT=1/(2*nn)*log(cosh(nn*(T+Tp-Ts))/cosh(nn*(T-Tp-Ts)))+Ts;

== matlab function Q0107tsmc_egtsmc_egftsmc_final_sensitivity/MATLAB Function20 ==
  data: Tmax input; TT output; Tmin input; nn input; T input
function TT = fcn(Tmax,Tmin,nn,T)
Ts=(Tmax+Tmin)/2;
Tp=(Tmax-Tmin)/2;
TT=1/(2*nn)*log(cosh(nn*(T+Tp-Ts))/cosh(nn*(T-Tp-Ts)))+Ts;

== matlab function Q0107tsmc_egtsmc_egftsmc_final_sensitivity/XBB3 ==
  data: ddxd input; dxd input; xd input; dxB input; xBB output; xB input
function xBB  = fcn(ddxd,dxd,xd,dxB,xB)


xBB=[ddxd',dxd',xd',dxB',xB'];

end

== matlab function Q0107tsmc_egtsmc_egftsmc_final_sensitivity/lambc4 ==
  data: Lp1 input; Lp2 input; Lp3 input; L1 input; L2 input; L3 input; f10 input; f11 input; f20 input; f21 input; f30 input; f31 input; rhos0 input; rhos1 input; rhos2 input; rhos3 input; rhos4 input; rhos5 input; rhos6 input; rhos7 input; rhos8 input; rhos9 input; rhos10 input; rhos11 input; p0 input; d10 input; d11 input; d20 input; d21 input; d30 input; d31 input; Os output size=[3 1]; U output; Uf input; bp1 output; bp2 output; bp3 output; bp4 output; bp5 output; bp6 output; bp7 output; bp8 output; bp9 output; bp10 output; bp11 output; bp12 output; lambc1 output; lambc2 output; lambc3 output; lambs1 output; lambs2 output; lambs3 output
function [Os,U,bp1,bp2,bp3,bp4,bp5,bp6,bp7,bp8,bp9,bp10,bp11,bp12,lambc1,lambc2,lambc3,lambs1,lambs2,lambs3]= fcn(Lp1,Lp2,Lp3,L1,L2,L3,f10,f11,f20,f21,f30,f31, ...
    rhos0,rhos1,rhos2,rhos3,rhos4,rhos5,rhos6,rhos7,rhos8,rhos9,rhos10,rhos11,p0,d10,d11,d20,d21,d30,d31,Uf)

bp1=f11*p0+f10-(rhos1*p0+rhos0)*L1-(rhos3*p0+rhos2)*L1*L1;
bp2=f21*p0+f20-(rhos5*p0+rhos4)*L2-(rhos7*p0+rhos6)*L2*L2;
bp3=f31*p0+f30-(rhos9*p0+rhos8)*L3-(rhos11*p0+rhos10)*L3*L3;
bp4=d11*p0+d10;
bp5=d21*p0+d20;
bp6=d31*p0+d30;
bp7=rhos1*p0+rhos0+2*L1*(rhos3*p0+rhos2);
bp8=rhos5*p0+rhos4+2*L2*(rhos7*p0+rhos6);
bp9=rhos9*p0+rhos8+2*L3*(rhos11*p0+rhos10);
bp10=rhos3*p0+rhos2;
bp11=rhos7*p0+rhos6;
bp12=rhos11*p0+rhos10;


lambc1 = rhos1*Lp1-rhos3*(Lp1*Lp1-2*L1*Lp1);
lambc2 = rhos5*Lp2-rhos7*(Lp2*Lp2-2*L2*Lp2);
lambc3 = rhos9*Lp3-rhos11*(Lp3*Lp3-2*L3*Lp3);

B1 = [lambc1 0 0 ;
    0 lambc2 0 ;
    0 0 lambc3];

lambs1 = f11-rhos1*L1-rhos3*L1*L1;
lambs2 = f21-rhos5*L2-rhos7*L2*L2;
lambs3 = f31-rhos9*L3-rhos11*L3*L3;

B2 = [-lambs1 0 0 ;
    0 -lambs2 0 ;
    0 0 -lambs3 ];


U = pinv(B2)*Uf;

Os = B1*U;



end

== matlab function Q0107tsmc_egtsmc_egftsmc_final_sensitivity/pso-RBF神经网络4/MATLAB Function14 ==
  data: c input; y output
function y = fcn(c)

y = [c;c;c];

== matlab function Q0107tsmc_egtsmc_egftsmc_final_sensitivity/pso-RBF神经网络4/MATLAB Function16 ==
  data: x input; y output
function y = fcn(x)

y = [-x -2*x/3 -x/3 0 x/3 x*2/3 x;
     -x -2*x/3 -x/3 0 x/3 x*2/3 x;
     -x -2*x/3 -x/3 0 x/3 x*2/3 x;
     -x -2*x/3 -x/3 0 x/3 x*2/3 x;
     -x -2*x/3 -x/3 0 x/3 x*2/3 x];

== matlab function Q0107tsmc_egtsmc_egftsmc_final_sensitivity/pso-RBF神经网络4/MATLAB Function7 ==
  data: c input; phix output; b input; x input
function phix = fcn(c,b,x)

phix=zeros(7,1);

for j = 1:1:7
     phix(j) = exp(-norm(x-c(:,j))^2/(b^2));  
end

== matlab function Q0107tsmc_egtsmc_egftsmc_final_sensitivity/pso-RBF神经网络4/MATLAB Function8 ==
  data: phix input; dgujiw output; k input; s input; Mf input
function dgujiw = fcn(phix,k,s,Mf)
dgujiw=zeros(3,7);
dgujiw=(k*phix*s'*pinv(Mf))';

== matlab function Q0107tsmc_egtsmc_egftsmc_final_sensitivity/滑模面4 ==
  data: e input; s output; de input; ie input; A input; B input; C input; gam1 input; gam2 input; rous output
function [s,rous]= fcn(e,de,ie,A,B,C,gam1,gam2)



s1=tanh(e(1))+A*abs(tanh(e(1)))^gam1*sign(e(1))+B*(1-(tanh(e(1))^2))^gam2*abs(de(1))^gam2*sign(de(1));
s2=tanh(e(2))+A*abs(tanh(e(2)))^gam1*sign(e(2))+B*(1-(tanh(e(2))^2))^gam2*abs(de(2))^gam2*sign(de(2));
s3=tanh(e(3))+A*abs(tanh(e(3)))^gam1*sign(e(3))+B*(1-(tanh(e(3))^2))^gam2*abs(de(3))^gam2*sign(de(3));

rous1=gam2*B*(1-tanh(e(1))^2)^gam2*abs(de(1))^(gam2-1);
rous2=gam2*B*(1-tanh(e(2))^2)^gam2*abs(de(2))^(gam2-1);
rous3=gam2*B*(1-tanh(e(3))^2)^gam2*abs(de(3))^(gam2-1);

rous=[rous1;rous2;rous3];


s=[s1;
   s2;
   s3];

== matlab function Q0107tsmc_egtsmc_egftsmc_final_sensitivity/MATLAB Function28 ==
  data: u input; out output; timeStepIdx input
function out = fcn(u, timeStepIdx)
    %#codegen
    
    % u 是输入的 200x3 矩阵
    % timeStepIdx 是当前时间步索引 (从外部提供，例如通过一个计数器)
    
    % 注意：如果计数器从0开始，则需要加1以符合MATLAB的1基索引
    adjustedTimeStepIdx = timeStepIdx + 1;
    
    % 获取原始数据的总行数
    num_rows = size(u, 1);
    
    % 检查索引是否超出范围
    if adjustedTimeStepIdx < 1 || adjustedTimeStepIdx > 2000
        error('Index out of bounds');
    end
    
    % 判断当前索引是否在原始数据范围内
    if adjustedTimeStepIdx <= num_rows
        % 如果在范围内，输出对应的数据行
        out = (u(adjustedTimeStepIdx, :));
        %out = rad2deg(u(adjustedTimeStepIdx, :));
    else
        % 如果超出范围，输出最后一行
        out = (u(num_rows, :));
        %out = rad2deg(u(num_rows, :));
    end

== matlab function Q0107tsmc_egtsmc_egftsmc_final_sensitivity/MATLAB Function29 ==
  data: phi1dd input; phi2dd input; Lp1d output; phi3dd input; alpha1 input; alpha2 input; alpha3 input; r input; Lx1 input; Lx2 input; Lx3 input; Lp2d output; Lp3d output
function [Lp1d,Lp2d,Lp3d]= fcn(phi1dd,phi2dd,phi3dd,alpha1,alpha2,alpha3,r,Lx1,Lx2,Lx3)





cos_term1 = cos(alpha1 - phi1dd);
Lp1d = sqrt(r^2 + Lx1^2 - 2 * r * Lx1 * cos_term1);

% 计算 Lp2d
cos_term2 = cos(alpha2 - phi2dd);
Lp2d = sqrt(r^2 + Lx2^2 - 2 * r * Lx2 * cos_term2);

% 计算 Lp3d
cos_term3 = cos(alpha3 - phi3dd);
Lp3d = sqrt(r^2 + Lx3^2 - 2 * r * Lx3 * cos_term3);
